simulink model "exp2_2019a"  (R2019a)
settings: Solver=ode1  StartTime=0.0  StopTime=20  FixedStep=0.001  MaxStep=0.01  RelTol=1e-3  AbsTol=1e-3  EnableMultiTasking=on
values from neighbouring files (symbols this model uses):
  a_1 = evalin('base','a_1')    [position.m]    (also in velocity.m)
  a_2 = evalin('base','a_2')    [position.m]    (also in velocity.m)
  a_3 = evalin('base','a_3')    [position.m]    (also in velocity.m)
  b_0 = evalin('base','b_0')    [position.m]    (also in velocity.m)
  b_1 = evalin('base','b_1')    [position.m]    (also in velocity.m)
  b_2 = evalin('base','b_2')    [position.m]    (also in velocity.m)
  b_3 = evalin('base','b_3')    [position.m]    (also in velocity.m)
  I_0 = evalin('base','I_0')    [position.m]    (also in velocity.m)
  I_1 = evalin('base','I_0')    [position.m]    (also in velocity.m)
  I_2 = evalin('base','I_0')    [position.m]    (also in velocity.m)
  I_3 = evalin('base','I_0')    [position.m]    (also in velocity.m)
  l_1 = evalin('base','l_1')    [position.m]    (also in velocity.m)
  l_2 = evalin('base','l_2')    [position.m]    (also in velocity.m)
  l_3 = evalin('base','l_3')    [position.m]    (also in velocity.m)
  M = evalin('base','M')    [position.m]    (also in velocity.m)
  m_0 = evalin('base','m_0')    [position.m]    (also in velocity.m)
  m_1 = evalin('base','m_1')    [position.m]    (also in velocity.m)
  m_2 = evalin('base','m_2')    [position.m]    (also in velocity.m)
  m_3 = evalin('base','m_3')    [position.m]    (also in velocity.m)
undefined symbols (not defined in the file or in its folder): X, Y, Z
libraries: sm_lib x33, nesl_utility x12
(part 2 of 2)

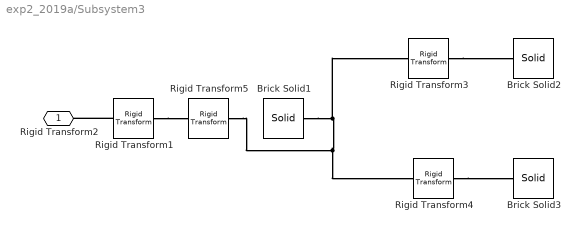
== system exp2_2019a/Subsystem3 ==
  Brick Solid1 : sm_lib/Body Elements/Solid  GraphicAmbientColor=[0.15 0.15 0.15 1.0]  BasedOnType=Mass  BrickDimensions=[L W R]  BrickDimensionUnits=m  CenterOfMass=[0 0 0]  CenterOfMassUnits=m  GraphicDiffuseColor=rgb  Density=1000  DensityUnits=kg/m^3  DoExposeReferenceFrame=on  GraphicEmissiveColor=[0.0 0.0 0.0 1.0]  ExportEntireGeometry=off  SerializedFrames=<Frames/>  MarkerShape=Sphere  MarkerSize=10  GraphicType=FromGeometry  InertiaType=CalculateFromGeometry  Mass=M  MassUnits=kg  MomentsOfInertia=[1 1 1]  MomentsOfInertiaUnits=kg*m^2  GraphicOpacity=1.0  ProductsOfInertia=[0 0 0]  ProductsOfInertiaUnits=kg*m^2  GraphicShininess=75  GraphicSpecularColor=[0.5 0.5 0.5 1.0]  GraphicVisPropType=SimpleVisualProperties  GeometryShape=Brick
  Brick Solid2 : sm_lib/Body Elements/Solid  GraphicAmbientColor=[0.15 0.15 0.15 1.0]  BasedOnType=Mass  BrickDimensions=[Ls Ws Rs]  BrickDimensionUnits=m  CenterOfMass=[0 0 0]  CenterOfMassUnits=m  GraphicDiffuseColor=rgb  Density=1000  DensityUnits=kg/m^3  DoExposeReferenceFrame=on  GraphicEmissiveColor=[0.0 0.0 0.0 1.0]  ExportEntireGeometry=off  SerializedFrames=<Frames/>  MarkerShape=Sphere  MarkerSize=10  GraphicType=FromGeometry  InertiaType=CalculateFromGeometry  Mass=M  MassUnits=kg  MomentsOfInertia=[1 1 1]  MomentsOfInertiaUnits=kg*m^2  GraphicOpacity=1.0  ProductsOfInertia=[0 0 0]  ProductsOfInertiaUnits=kg*m^2  GraphicShininess=75  GraphicSpecularColor=[0.5 0.5 0.5 1.0]  GraphicVisPropType=SimpleVisualProperties  GeometryShape=Brick
  Brick Solid3 : sm_lib/Body Elements/Solid  GraphicAmbientColor=[0.15 0.15 0.15 1.0]  BasedOnType=Mass  BrickDimensions=[Ls Ws Rs]  BrickDimensionUnits=m  CenterOfMass=[0 0 0]  CenterOfMassUnits=m  GraphicDiffuseColor=rgb  Density=1000  DensityUnits=kg/m^3  DoExposeReferenceFrame=on  GraphicEmissiveColor=[0.0 0.0 0.0 1.0]  ExportEntireGeometry=off  SerializedFrames=<Frames/>  MarkerShape=Sphere  MarkerSize=10  GraphicType=FromGeometry  InertiaType=CalculateFromGeometry  Mass=M  MassUnits=kg  MomentsOfInertia=[1 1 1]  MomentsOfInertiaUnits=kg*m^2  GraphicOpacity=1.0  ProductsOfInertia=[0 0 0]  ProductsOfInertiaUnits=kg*m^2  GraphicShininess=75  GraphicSpecularColor=[0.5 0.5 0.5 1.0]  GraphicVisPropType=SimpleVisualProperties  GeometryShape=Brick
  Rigid Transform1 : sm_lib/Frames and Transforms/Rigid Transform  TranslationMethod=StandardAxis  TranslationStandardOffset=R/2  TranslationLengthUnit=m  TranslationStandardAxis=+X  TranslationCartesianOffset=[0 0 0]  TranslationROffset=0  TranslationROffsetUnits=m  TranslationZOffset=0  TranslationZOffsetUnits=m  TranslationThetaOffset=0  TranslationThetaOffsetUnits=deg  RotationMethod=None  RotationAngleUnits=deg  RotationStandardAxis=+Z  RotationAngle=0.0  RotationArbitraryAxis=[0 0 1]  FollAlignAxisA=+X  BaseAlignAxisA=+Y  FollAlignAxisB=+Y  BaseAlignAxisB=+Z  RotationSequenceAxes=FollowerAxes  RotationSequence=XYX  RotationSequenceAngles=[0 0 0]  RotationSequenceAnglesUnits=deg  RotationMatrix=[1 0 0; 0 1 0; 0 0 1]
  Rigid Transform3 : sm_lib/Frames and Transforms/Rigid Transform  TranslationMethod=Cartesian  TranslationStandardOffset=L  TranslationLengthUnit=m  TranslationStandardAxis=-X  TranslationCartesianOffset=[-L W/2 0]  TranslationROffset=0  TranslationROffsetUnits=m  TranslationZOffset=0  TranslationZOffsetUnits=m  TranslationThetaOffset=0  TranslationThetaOffsetUnits=deg  RotationMethod=None  RotationAngleUnits=deg  RotationStandardAxis=+Z  RotationAngle=0.0  RotationArbitraryAxis=[0 0 1]  FollAlignAxisA=+X  BaseAlignAxisA=+Y  FollAlignAxisB=+Y  BaseAlignAxisB=+Z  RotationSequenceAxes=FollowerAxes  RotationSequence=XYX  RotationSequenceAngles=[0 0 0]  RotationSequenceAnglesUnits=deg  RotationMatrix=[1 0 0; 0 1 0; 0 0 1]
  Rigid Transform4 : sm_lib/Frames and Transforms/Rigid Transform  TranslationMethod=Cartesian  TranslationStandardOffset=L  TranslationLengthUnit=m  TranslationStandardAxis=-X  TranslationCartesianOffset=[-L -W/2 0]  TranslationROffset=0  TranslationROffsetUnits=m  TranslationZOffset=0  TranslationZOffsetUnits=m  TranslationThetaOffset=0  TranslationThetaOffsetUnits=deg  RotationMethod=None  RotationAngleUnits=deg  RotationStandardAxis=+Z  RotationAngle=0.0  RotationArbitraryAxis=[0 0 1]  FollAlignAxisA=+X  BaseAlignAxisA=+Y  FollAlignAxisB=+Y  BaseAlignAxisB=+Z  RotationSequenceAxes=FollowerAxes  RotationSequence=XYX  RotationSequenceAngles=[0 0 0]  RotationSequenceAnglesUnits=deg  RotationMatrix=[1 0 0; 0 1 0; 0 0 1]
  Rigid Transform5 : sm_lib/Frames and Transforms/Rigid Transform  TranslationMethod=StandardAxis  TranslationStandardOffset=R/2  TranslationLengthUnit=m  TranslationStandardAxis=-X  TranslationCartesianOffset=[0 0 0]  TranslationROffset=0  TranslationROffsetUnits=m  TranslationZOffset=0  TranslationZOffsetUnits=m  TranslationThetaOffset=0  TranslationThetaOffsetUnits=deg  RotationMethod=StandardAxis  RotationAngleUnits=deg  RotationStandardAxis=+Z  RotationAngle=180  RotationArbitraryAxis=[0 0 1]  FollAlignAxisA=+X  BaseAlignAxisA=+Y  FollAlignAxisB=+Y  BaseAlignAxisB=+Z  RotationSequenceAxes=FollowerAxes  RotationSequence=XYX  RotationSequenceAngles=[0 0 0]  RotationSequenceAnglesUnits=deg  RotationMatrix=[1 0 0; 0 1 0; 0 0 1]
  Rigid Transform2 : PMIOPort  Side=Left
  connections:
  Brick Solid1/RConn1 -- Rigid Transform5/RConn1 -- Rigid Transform4/LConn1 -- Rigid Transform3/LConn1
  Rigid Transform1/LConn1 -- Rigid Transform2/RConn1
  Rigid Transform3/RConn1 -- Brick Solid2/RConn1
  Rigid Transform4/RConn1 -- Brick Solid3/RConn1
  Rigid Transform1/RConn1 -- Rigid Transform5/LConn1

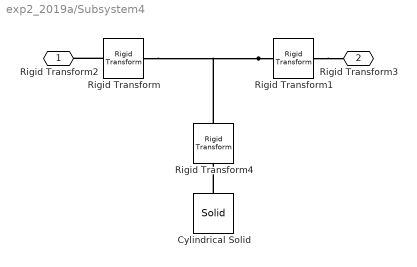
== system exp2_2019a/Subsystem4 ==
  Cylindrical Solid : sm_lib/Body Elements/Solid  GraphicAmbientColor=[0.15 0.15 0.15 1.0]  BasedOnType=Mass  CenterOfMass=[0 0 0]  CenterOfMassUnits=m  GraphicDiffuseColor=rgb  CylinderLength=L  CylinderLengthUnits=m  CylinderRadius=R  CylinderRadiusUnits=m  Density=1000  DensityUnits=kg/m^3  DoExposeReferenceFrame=on  GraphicEmissiveColor=[0.0 0.0 0.0 1.0]  ExportEntireGeometry=off  SerializedFrames=<Frames/>  MarkerShape=Sphere  MarkerSize=10  GraphicType=FromGeometry  InertiaType=CalculateFromGeometry  Mass=M  MassUnits=kg  MomentsOfInertia=[1 1 1]  MomentsOfInertiaUnits=kg*m^2  GraphicOpacity=1.0  ProductsOfInertia=[0 0 0]  ProductsOfInertiaUnits=kg*m^2  GraphicShininess=75  GraphicSpecularColor=[0.5 0.5 0.5 1.0]  GraphicVisPropType=SimpleVisualProperties  GeometryShape=Cylinder
  Rigid Transform : sm_lib/Frames and Transforms/Rigid Transform  TranslationMethod=StandardAxis  TranslationStandardOffset=L/2  TranslationLengthUnit=m  TranslationStandardAxis=-X  TranslationCartesianOffset=[0 0 0]  TranslationROffset=0  TranslationROffsetUnits=m  TranslationZOffset=0  TranslationZOffsetUnits=m  TranslationThetaOffset=0  TranslationThetaOffsetUnits=deg  RotationMethod=None  RotationAngleUnits=deg  RotationStandardAxis=+Z  RotationAngle=0.0  RotationArbitraryAxis=[0 0 1]  FollAlignAxisA=+X  BaseAlignAxisA=+Y  FollAlignAxisB=+Y  BaseAlignAxisB=+Z  RotationSequenceAxes=FollowerAxes  RotationSequence=XYX  RotationSequenceAngles=[0 0 0]  RotationSequenceAnglesUnits=deg  RotationMatrix=[1 0 0; 0 1 0; 0 0 1]
      settings: SourceProductName=Multibody
  Rigid Transform1 : sm_lib/Frames and Transforms/Rigid Transform  TranslationMethod=StandardAxis  TranslationStandardOffset=L/2  TranslationLengthUnit=m  TranslationStandardAxis=+X  TranslationCartesianOffset=[0 0 0]  TranslationROffset=0  TranslationROffsetUnits=m  TranslationZOffset=0  TranslationZOffsetUnits=m  TranslationThetaOffset=0  TranslationThetaOffsetUnits=deg  RotationMethod=None  RotationAngleUnits=deg  RotationStandardAxis=+Z  RotationAngle=0.0  RotationArbitraryAxis=[0 0 1]  FollAlignAxisA=+X  BaseAlignAxisA=+Y  FollAlignAxisB=+Y  BaseAlignAxisB=+Z  RotationSequenceAxes=FollowerAxes  RotationSequence=XYX  RotationSequenceAngles=[0 0 0]  RotationSequenceAnglesUnits=deg  RotationMatrix=[1 0 0; 0 1 0; 0 0 1]
      settings: SourceProductName=Multibody
  Rigid Transform4 : sm_lib/Frames and Transforms/Rigid Transform  TranslationMethod=None  TranslationStandardOffset=0  TranslationLengthUnit=m  TranslationStandardAxis=+Z  TranslationCartesianOffset=[0 0 0]  TranslationROffset=0  TranslationROffsetUnits=m  TranslationZOffset=0  TranslationZOffsetUnits=m  TranslationThetaOffset=0  TranslationThetaOffsetUnits=deg  RotationMethod=StandardAxis  RotationAngleUnits=deg  RotationStandardAxis=+Y  RotationAngle=90  RotationArbitraryAxis=[0 0 1]  FollAlignAxisA=+X  BaseAlignAxisA=+Y  FollAlignAxisB=+Y  BaseAlignAxisB=+Z  RotationSequenceAxes=FollowerAxes  RotationSequence=XYX  RotationSequenceAngles=[0 0 0]  RotationSequenceAnglesUnits=deg  RotationMatrix=[1 0 0; 0 1 0; 0 0 1]
  Rigid Transform2 : PMIOPort  Side=Left
  Rigid Transform3 : PMIOPort  Port=2  Side=Right
  connections:
  Cylindrical Solid/RConn1 -- Rigid Transform4/LConn1
  Rigid Transform1/LConn1 -- Rigid Transform3/RConn1
  Rigid Transform/LConn1 -- Rigid Transform2/RConn1
  Rigid Transform1/RConn1 -- Rigid Transform4/RConn1 -- Rigid Transform/RConn1

== matlab function exp2_2019a/MATLAB Function ==
  data: r_0x input; v_0x output; r_0y input; theta_0 input; theta_1 input; theta_2 input; theta_3 input; theta_dot_1 input; theta_dot_2 input; theta_dot_3 input; v_0y output; w_0 output; v_ex output; v_ey output; w_e output; a_1 parameter; a_2 parameter; a_3 parameter; b_0 parameter; b_1 parameter; b_2 parameter; b_3 parameter; l_1 parameter; l_2 parameter; l_3 parameter; m_0 parameter; m_1 parameter; m_2 parameter; m_3 parameter; M parameter; I_0 parameter; I_1 parameter; I_2 parameter; I_3 parameter; J_g output
%通过公式6-363计算末端速度
function [v_0x,v_0y,w_0,v_ex,v_ey,w_e,J_g] = velocity(r_0x,r_0y,theta_0,theta_1,theta_2,theta_3,theta_dot_1,theta_dot_2,theta_dot_3, a_1, a_2, a_3, b_0, b_1, b_2, b_3, l_1, l_2, l_3, m_0, m_1, m_2, m_3, M, I_0, I_1, I_2, I_3)
    %读取工作空间的所有变量
%     a_1 = evalin('base','a_1');
%     a_2 = evalin('base','a_2');
%     a_3 = evalin('base','a_3');
%     b_0 = evalin('base','b_0');
%     b_1 = evalin('base','b_1');
%     b_2 = evalin('base','b_2');
%     b_3 = evalin('base','b_3');
%     l_1 = evalin('base','l_1');
%     l_2 = evalin('base','l_2');
%     l_3 = evalin('base','l_3');
%     m_0 = evalin('base','m_0');
%     m_1 = evalin('base','m_1');
%     m_2 = evalin('base','m_2');
%     m_3 = evalin('base','m_3');
%     M = evalin('base','M');
%     I_0 = evalin('base','I_0');
%     I_1 = evalin('base','I_0');
%     I_2 = evalin('base','I_0');
%     I_3 = evalin('base','I_0');

    %更新各个参量
    s_0 = sin(theta_0);
    c_0 = cos(theta_0);
    s_01 = sin(theta_0+theta_1);
    c_01 = cos(theta_0+theta_1);
    s_012 = sin(theta_0+theta_1+theta_2);
    c_012 = cos(theta_0+theta_1+theta_2);
    s_0123 = sin(theta_0+theta_1+theta_2+theta_3);
    c_0123 = cos(theta_0+theta_1+theta_2+theta_3);

    k_vx = -m_1*(b_0*s_0+a_1*s_01)-m_2*(b_0*s_0+l_1*s_01+a_2*s_012)-m_3*(b_0*s_0+l_1*s_01+l_2*s_012+a_3*s_0123); %公式6-321    check
    k_vy = m_1*(b_0*c_0+a_1*c_01)+m_2*(b_0*c_0+l_1*c_01+a_2*c_012)+m_3*(b_0*c_0+l_1*c_01+l_2*c_012+a_3*c_0123); %公式6-322     check
    k_px1 = -m_1*a_1*s_01-m_2*(l_1*s_01+a_2*s_012)-m_3*(l_1*s_01+l_2*s_012+a_3*s_0123);%公式6-323   check
    k_px2 = -m_2*a_2*s_012 - m_3*(l_2*s_012+a_3*s_0123); %公式6-324   check
    k_px3 = -m_3*a_3*s_0123; %公式6-325    check

    k_py1 = m_1*a_1*c_01+m_2*(l_1*c_01+a_2*c_012)+m_3*(l_1*c_01+l_2*c_012+a_3*c_0123); %公式6-326   check
    k_py2 = m_2*a_2*c_012+m_3*(l_2*c_012+a_3*c_0123);  %公式6-327   check
    k_py3 = m_3*a_3*c_0123;  %公式6-328  check

    k_w = (I_0+I_1+I_2+I_3) + m_1*(b_0*c_0+a_1*c_01)^2 +m_1*(b_0*s_0+a_1*s_01)^2 ...
        +m_2*(b_0*c_0+l_1*c_01+a_2*c_012)^2+m_2*(b_0*s_0+l_1*s_01+a_2*s_012)^2 ...
        +m_2*(b_0*c_0+l_1*c_01+l_2*c_012+a_3*c_0123)^2 + m_3*(b_0*s_0+l_1*s_01+l_2*s_012+a_3*s_0123)^2 ...
        -M*(r_0x^2+r_0y^2); %公式6-353   check

    k_q1 = (I_1+I_2+I_3) +m_1*a_1*c_01*(b_0*c_0+a_1*c_01)+m_1*a_1*s_01*(b_0*s_0+a_1*s_01) ...
        +m_2*(l_1*c_01+a_2*c_012)*(b_0*c_0+l_1*c_01+a_2*c_012) ...
        +m_2*(l_1*s_01+a_2*s_012)*(b_0*s_0+l_1*s_01+a_2*s_012) ...
        +m_3*(l_1*c_01+l_2*c_012+a_3*c_0123)*(b_0*c_0+l_1*c_01+l_2*c_012+a_3*c_0123) ...
        +m_3*(l_1*s_01+l_2*s_012+a_3*s_0123)*(b_0*s_0+l_1*s_01+l_2*s_012+a_3*s_0123) ...
        +r_0x*(m_1*a_1*c_01+m_2*(l_1*c_01+a_2*c_012)+m_3*(l_1*c_01+l_2*c_012+a_3*c_0123)) ...
        +r_0y*(m_1*a_1*s_01+m_2*(l_1*s_01+a_2*s_012)+m_3*(l_1*s_01+l_2*s_012+a_3*s_0123)); %公式6-354    check

    k_q2 = (I_2+I_3)+m_2*a_2*c_012*(b_0*c_0+l_1*c_01+a_2*c_012)+m_2*a_2*s_012*(b_0*s_0+l_1*s_01+a_2*s_012) ...
        +m_3*(l_2*c_012+a_3*c_0123)*(b_0*c_0+l_1*c_01+l_2*c_012+a_3*c_0123) ...
        +m_3*(l_2*s_012+a_3*s_0123)*(b_0*s_0+l_1*s_01+l_2*s_012+a_3*s_0123) ...
        +r_0x*(m_2*a_2*c_012+m_3*(l_2*c_012+a_3*c_0123)) ...
        +r_0y*(m_2*a_2*s_012+m_3*(l_2*s_012+a_3*s_0123));%公式6-355     check

    k_q3 = I_3+m_3*a_3*c_0123*(b_0*c_0+l_1*c_01+l_2*c_012+a_3*c_0123)+m_3*a_3*s_0123*(b_0*s_0+l_1*s_01+l_2*s_012+a_3*s_0123) ...
        +m_3*a_3*c_0123*r_0x+m_3*a_3*s_0123*r_0y;%公式6-356     check

    J_s = [
        1     0     -b_0*s_0-l_1*s_01-l_2*s_012-l_3*s_0123;
        0     1      b_0*c_0+l_1*c_01+l_2*c_012+l_3*c_0123;
        0     0                        1                  ;
        ];%公式6-309   check
    J_m = [
        -l_1*s_01-l_2*s_012-l_3*s_0123  -l_2*s_012-l_3*s_0123    -l_3*s_0123;
         l_1*c_01+l_2*c_012+l_3*c_0123   l_2*c_012+l_3*c_0123     l_3*c_0123;
         1                               1                        1         ;
        ];  %公式6-310  check

    J_1 = [
        M   0   k_vx;
        0   M   k_vy;
        0   0   k_w ;
        ];%公式6-360  check
    J_2 = [
        k_px1  k_px2  k_px3;
        k_py1  k_py2  k_py3;
        k_q1   k_q2   k_q3
        ];%公式6-361   check
    J_g = -J_s*inv(J_1)*J_2+J_m;  %公式6-363  check

    
    %计算速度
    velocity_end = J_g*[theta_dot_1;theta_dot_2;theta_dot_3]; %末端速度
    velocity_0 = -inv(J_1)*J_2*[theta_dot_1;theta_dot_2;theta_dot_3];%基座速度
    v_ex = velocity_end(1);
    v_ey = velocity_end(2);
    w_e = velocity_end(3);
    v_0x = velocity_0(1);
    v_0y = velocity_0(2);
    w_0 = velocity_0(3);

== matlab function exp2_2019a/MATLAB Function2 ==
  data: theta_0 input; r_0x output; theta_1 input; theta_2 input; theta_3 input; r_0y output; p_ex output; p_ey output; Phi_e output; a_1 parameter; a_2 parameter; a_3 parameter; b_0 parameter; b_1 parameter; b_2 parameter; b_3 parameter; l_1 parameter; l_2 parameter; l_3 parameter; m_0 parameter; m_1 parameter; m_2 parameter; m_3 parameter; M parameter; I_0 parameter; I_1 parameter; I_2 parameter; I_3 parameter
%根据公式6-294和6-295,6-296进行建模
function [r_0x,r_0y,p_ex,p_ey,Phi_e] = position(theta_0,theta_1,theta_2,theta_3, a_1, a_2, a_3, b_0, b_1, b_2, b_3, l_1, l_2, l_3, m_0, m_1, m_2, m_3, M, I_0, I_1, I_2, I_3)
    %读取工作空间的所有变量
%     a_1
%     a_1 = evalin('base','a_1');
%     a_2 = evalin('base','a_2');
%     a_3 = evalin('base','a_3');
%     b_0 = evalin('base','b_0');
%     b_1 = evalin('base','b_1');
%     b_2 = evalin('base','b_2');
%     b_3 = evalin('base','b_3');
%     l_1 = evalin('base','l_1');
%     l_2 = evalin('base','l_2');
%     l_3 = evalin('base','l_3');
%     m_0 = evalin('base','m_0');
%     m_1 = evalin('base','m_1');
%     m_2 = evalin('base','m_2');
%     m_3 = evalin('base','m_3');
%     M = evalin('base','M');
%     I_0 = evalin('base','I_0');
%     I_1 = evalin('base','I_0');
%     I_2 = evalin('base','I_0');
%     I_3 = evalin('base','I_0');
    
    %计算参数
    s_0 = sin(theta_0);
    c_0 = cos(theta_0);
    s_01 = sin(theta_0+theta_1);
    c_01 = cos(theta_0+theta_1);
    s_012 = sin(theta_0+theta_1+theta_2);
    c_012 = cos(theta_0+theta_1+theta_2);
    s_0123 = sin(theta_0+theta_1+theta_2+theta_3);
    c_0123 = cos(theta_0+theta_1+theta_2+theta_3);
    
    b_0_hat = m_0/M*b_0;
    b_1_hat = (m_0 + m_1)/M*b_1;
    b_2_hat = (m_0 + m_1 + m_2)/M*b_2;
    b_3_hat = b_2;

    a_1_hat = m_0/M*a_1;
    a_2_hat = (m_0+m_1)/M*a_2;
    a_3_hat = (m_0+m_1+m_2)/M*a_3;
    
    %计算r_0 公式6-293  check
    r_0x = -( (m_1+m_2+m_3)/M*b_0*c_0 + ((m_1+m_2+m_3)/M*a_1 + (m_2+m_3)/M*b_1)*c_01 + ((m_2+m_3)/M*a_2 + m_3/M*b_2)*c_012 + m_3/M*a_3*c_0123);
    r_0y = -( (m_1+m_2+m_3)/M*b_0*s_0 + ((m_1+m_2+m_3)/M*a_1 + (m_2+m_3)/M*b_1)*s_01 + ((m_2+m_3)/M*a_2 + m_3/M*b_2)*s_012 + m_3/M*a_3*s_0123);
    
    
    %计算末端位姿
    p_ex = b_0_hat*c_0 + (a_1_hat+b_1_hat)*c_01 + (a_2_hat+b_2_hat)*c_012+(a_3_hat+b_3_hat)*c_0123;
    p_ey = b_0_hat*s_0 + (a_1_hat+b_1_hat)*s_01 + (a_2_hat+b_2_hat)*s_012+(a_3_hat+b_3_hat)*s_0123;
    Phi_e = theta_0+theta_1+theta_2+theta_3;%末端姿态角

== matlab function exp2_2019a/MATLAB Function3 ==
  data: u input; theta_1_dot output; p_e0 input; p_ef input; phi_e0 input; phi_ef input; tf input; ts input; J_g input; theta_2_dot output; theta_3_dot output; v_ex_plan output; v_ey_plan output; w_e_plan output; det_J output; det_Jg output
function [theta_1_dot,theta_2_dot,theta_3_dot,v_ex_plan,v_ey_plan,w_e_plan,det_J,det_Jg] = path_plan_continue(u,p_e0,p_ef,phi_e0,phi_ef, tf, ts, J_g)
%使用11.7.1章中的笛卡尔空间连续位姿跟踪的方法进行规划
    
    v_em = (p_ef-p_e0)/(tf-ts); %速度最大值
    
    w_em = (phi_ef-phi_e0)/(tf-ts); %角速度最大值
    
    %按照梯形函数输出
    
    if(u<ts)
        v_e = v_em/ts*u;
        w_e = w_em/ts*u;
    elseif(u < tf-ts)
        v_e = v_em;
        w_e = w_em;
        
    else
        v_e = v_em-v_em/ts*(u-tf+ts);
        w_e = w_em-w_em/ts*(u-tf+ts);
    end

    v_ex = v_e(1);
    v_ey = v_e(2);
    u
    J_g
    % 防止奇异
    J = J_g;
%     %奇异值分解
%     s = svd(J); % 降序返回矩阵J的奇异值
%     lamda_m = 0.5;
%     epsilon = 0.0001;%是否为奇异的判定条件
%     if(s(3)>epsilon)
%         lamda_2 = 0;
%     else
%         lamda_2 = (1-(s(3)/epsilon)^2)*lamda_m^2;
%     end
%     J = J_g'/(J_g*J_g'+lamda_2*eye(size(J_g)));

    
    %防止初始时刻J_g是零矩阵导致的错误
    if(det(J)==0)
        theta_1_dot=0;
        theta_2_dot=0;
        theta_3_dot=0;
    else
        theta_dot = J\[v_ex,v_ey,w_e]';
        theta_1_dot = theta_dot(1);
        theta_2_dot = theta_dot(2);
        theta_3_dot = theta_dot(3);
    end
    det_J = cond(J);
    det_Jg = det(J_g);
    v_ex_plan = v_ex;
     
    v_ey_plan = v_ey;
    w_e_plan = w_e;
    




end
